simulink library "Hydraulic_Actuator_Lib"  (Simulink 7.9)
settings: Solver=ode45  StartTime=0.0  StopTime=10.0  RelTol=1e-3
undefined symbols (not defined in the file or in its folder): WT_Params
libraries: fl_lib x20, nesl_utility x10, sh_lib x9, mblibv1 x1
Description:
  | Copyright 2011 MathWorks, Inc.
settings Model: Creator=smiller  LastModifiedBy=smiller

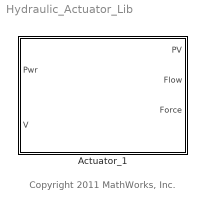
== system Hydraulic_Actuator_Lib ==
  note: Copyright 2011 MathWorks, Inc.
  Actuator_1 : Subsystem
      mask Display: image(imread('Pitch_Hydraulic_Actuator_IMAGE.jpg'));

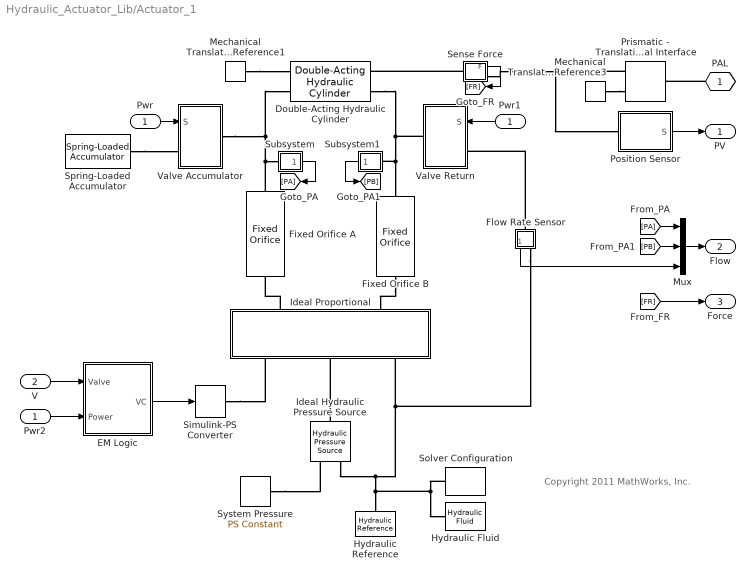
== system Hydraulic_Actuator_Lib/Actuator_1 ==
  note: Copyright 2011 MathWorks, Inc.
  Pwr : Inport
  V : Inport  Port=2
  Double-Acting Hydraulic Cylinder : sh_lib/Hydraulic Cylinders/Double-Acting Hydraulic Cylinder  SystemSampleTime=-1  area_A=WT_Params.Pitch_Actuator.Cylinder.piston_area m^2  area_B=WT_Params.Pitch_Actuator.Cylinder.piston_area m^2  stroke=WT_Params.Pitch_Actuator.Cylinder.stroke m  init_pos=WT_Params.Pitch_Actuator.Cylinder.initial_disp_from_a m  dead_vol_A=1e-04 m^3  dead_vol_B=1e-04 m^3  init_pressure_A=0 Pa  init_pressure_B=0 Pa  k_sh=1.4  stiff=WT_Params.Pitch_Actuator.Cylinder.contact_stiffness N/m  D=WT_Params.Pitch_Actuator.Cylinder.contact_damping N/(m/s)  or=2  LocalVarLogging=[]
  EM Logic : Subsystem
  Fixed Orifice A : sh_lib/Orifices/Fixed Orifice  SystemSampleTime=-1  area=WT_Params.Pitch_Actuator.orifice_area m^2  C_d=0.7  Re_cr=12  flow_rate_Log=off  pr_drop_Log=off  Re_Log=off  power_Log=off  LocalVarNames=|flow_rate|pr_drop|Re|power  LocalVarDescs=|Flow rate through the orifice (m^3/s)|Pressure drop across the orifice (Pa)|Reynolds number|Power (W)  LocalVarLogging=[0 0 0 0]
  Fixed Orifice B : sh_lib/Orifices/Fixed Orifice  SystemSampleTime=-1  area=WT_Params.Pitch_Actuator.orifice_area m^2  C_d=0.7  Re_cr=12  flow_rate_Log=off  pr_drop_Log=off  Re_Log=off  power_Log=off  LocalVarNames=|flow_rate|pr_drop|Re|power  LocalVarDescs=|Flow rate through the orifice (m^3/s)|Pressure drop across the orifice (Pa)|Reynolds number|Power (W)  LocalVarLogging=[0 0 0 0]
  Flow Rate Sensor : Subsystem
      mask Display: disp('F')
  Hydraulic Reference : fl_lib/Hydraulic/Hydraulic Elements/Hydraulic Reference  SystemSampleTime=-1  q_Log=off  LocalVarNames=|q  LocalVarDescs=|q  LocalVarLogging=[]
  Hydraulic Fluid : sh_lib/Hydraulic Utilities/Hydraulic Fluid  SystemSampleTime=-1  DataSource=1  SelFluid=1  SysTemp=60 c  TrapAir=0.005  ViscDerFactor=1  LocalVarLogging=[]
  Ideal Proportional : Subsystem
      mask Display:
      | plot([198.418507352471;198.418507352471], [5.66910021007061;25.5109509453177])
      | plot([189.914857037365;206.922157667577], [25.5109509453177;25.5109509453177])
      | plot([240.936758928001;240.936758928001], [5.66910021007061;25.5109509453177])
      | plot([232.433108612895;249.440409243107], [25.5109509453177;25.5109509453177])
      | plot([240.936758928001;240.936758928001], [76.5328528359532;56.6910021007061])
      | plot([232.433108612895;249.440409243107], [56.6910021007061;56.6910021007061])
      | plot([198.418507352471;198.418507352471], [76.5328528359532;56.6910021007061])
      | plot([189.914857037365;206.922157667577], [56.6910021007061;56.6910021007061])
      | plot([99.2092536762357;99.2092536762357], [76.5328528359532;5.66910021007061])
      | plot([141.727505251765;141.727505251765], [76.5328528359532;5.66910021007061])
      | plot([170.073006302118;170.073006302118], [76.5328528359532;5.66910021007061])
      | plot([269.282259978354;269.282259978354], [76.5328528359532;5.66910021007061])
      | patch([99.2092536762357;93.5401534661651;104.878353886306;99.2092536762357], [76.5328528359532;53.8564519956708;53.8564519956708;76.5328528359532],[0 0 0])
      | plot([99.2092536762357;93.5401534661651;104.878353886306;99.2092536762357], [76.5328528359532;53.8564519956708;53.8564519956708;76.5328528359532])
      | patch([141.727505251765;136.058405041695;147.396605461836;141.727505251765], [5.66910021007061;28.3455010503531;28.3455010503531;5.66910021007061],[0 0 0])
      | plot([141.727505251765;136.058405041695;147.396605461836;141.727505251765], [5.66910021007061;28.3455010503531;28.3455010503531;5.66910021007061])
      | plot([297.627761028707;340.146012604237], [5.66910021007061;76.5328528359532])
      | plot([297.627761028707;340.146012604237], [76.5328528359532;5.66910021007061])
      | plot([70.8637526258826;368.49151365459;368.49151365459;70.8637526258826;70.8637526258826], [76.5328528359532;76.5328528359532;5.66910021007061;5.66910021007061;76.5328528359532])
      | patch([297.627761028707;303.296861238778;311.800511553884;297.627761028707], [5.66910021007061;25.5109509453177;19.8418507352471;5.66910021007061],[0 0 0])
      | plot([297.627761028707;303.296861238778;311.800511553884;297.627761028707], [5.66910021007061;25.5109509453177;19.8418507352471;5.66910021007061])
      | patch([297.627761028707;303.296861238778;311.800511553884;297.627761028707], [76.5328528359532;56.6910021007061;62.3601023107767;76.5328528359532],[0 0 0])
      | plot([297.627761028707;303.296861238778;311.800511553884;297.627761028707], [76.5328528359532;56.6910021007061;62.3601023107767;76.5328528359532])
      | plot([62.3601023107767;374.16061386466], [82.2019530460238;82.2019530460238])
      | plot([65.194652415812;376.995163969696], [0;0])
      | plot([70.8637526258826;0;0;70.8637526258826;70.8637526258826], [53.8564519956708;53.8564519956708;25.5109509453177;25.5109509453177;53.8564519956708]-25.5109509453177+5.66910021007061)
      | plot([70.8637526258826;0;0;70.8637526258826;70.8637526258826]+368.49151365459, [53.8564519956708;53.8564519956708;25.5109509453177;25.5109509453177;53.8564519956708]-25.5109509453177+5.66910021007061)
      | plot([15 25], [5.66910021007061 35])
      | plot([25 15]+405, [5.66910021007061 35])
      | plot([42.5 40]+5,[70 58]);
      | plot([45 50]+2.5,[70 45]);
      | plot([45 50]+7.5,[45 70]);
      | plot([45 50]+12.5,[70 45]);
      | plot([45 50]+17.5,[45 70]);
      | plot([40 42.5]+27.5,[70 58]);
      | plot([42.5 40]+5+324,[70 58]);
      | plot([45 50]+2.5+324,[70 45]);
      | plot([45 50]+7.5+324,[45 70]);
      | plot([45 50]+12.5+324,[70 45]);
      | plot([45 50]+17.5+324,[45 70]);
      | plot([40 42.5]+27.5+324,[70 58]);
      | ;color('red');
      | port_label('LConn', 1,'A')
      | port_label('LConn', 2,'B')
      | port_label('RConn', 1,'S')
      | port_label('RConn', 2,'P')
      | port_label('RConn', 3,'T')
  Ideal Hydraulic Pressure Source : fl_lib/Hydraulic/Hydraulic Sources/Hydraulic Pressure Source  SystemSampleTime=-1  q_Log=off  p_Log=off  LocalVarNames=|flow_rate|pr_differential|power  LocalVarDescs=|Flow rate through the source (m^3/s)|Pressure differential across the source (Pa)|Source power (W)  LocalVarLogging=[0 0 0]
  Mechanical Translational Reference1 : fl_lib/Mechanical/Translational Elements/Mechanical Translational Reference  Tag=Factory Generic  SystemSampleTime=-1  f_Log=off  LocalVarNames=|f  LocalVarDescs=|f  LocalVarLogging=[]
  Mechanical Translational Reference3 : fl_lib/Mechanical/Translational Elements/Mechanical Translational Reference  Tag=Factory Generic  SystemSampleTime=-1  f_Log=off  LocalVarNames=|f  LocalVarDescs=|f  LocalVarLogging=[]
  Mux : Mux  Inputs=3
  Position Sensor : Subsystem
      mask Display:
      | plot([25.5109509453177;56.6910021007061;70.8637526258826;96.3747035712004;127.554754726589;155.900255776942;184.245756827295;212.591257877648;235.26765871793;252.274959348142;283.455010503531], [155.900255776942;155.900255776942;110.547454096377;198.418507352471;113.382004201412;198.418507352471;116.216554306448;198.418507352471;113.382004201412;155.900255776942;155.900255776942])
      | plot([155.900255776942;155.900255776942], [266.447709873319;198.418507352471])
      | patch([155.900255776942;170.073006302118;141.727505251765;155.900255776942], [198.418507352471;226.764008402824;226.764008402824;198.418507352471], [0;0;0])
      | plot([155.900255776942;170.073006302118;141.727505251765;155.900255776942], [198.418507352471;226.764008402824;226.764008402824;198.418507352471])
      | ;
      | color('red');
      | port_label('LConn', 1,'R')
      | port_label('output', 1,'P')
  Prismatic - Translational Interface : mblibv1/Interface  Elements/Prismatic - Translational Interface  UpdateFromCAD=off  DialogClass=PrismaticTranslationalInterface  Primitive=P1
  Pwr1 : InportShadow  Port=1
  Pwr2 : InportShadow  Port=1
  Sense Force : Subsystem
      mask Display: disp('F');
  Simulink-PS Converter : nesl_utility/Simulink-PS Converter  SystemSampleTime=-1  PhysicalDomain=network_engine_domain  LeftPortType=input  RightPortType=output  SubClassName=ps_input  Unit=1  AffineConversion=off  InputFilterTimeConstant=.001  UdotUserProvided=0
  Solver Configuration : nesl_utility/Solver Configuration  SystemSampleTime=-1  PhysicalDomain=network_engine_domain  LeftPortType=input  RightPortType=generic  SubClassName=solver  Accelerate=off  Profile=off  ResidualTolerance=WT_Params.Pitch_Actuator.constraint_tol  MaxNonlinIter=12  MaxModeIter=2  DoFixedCost=off  UseLocalSampling=off  DoDC=off  LinearAlgebra=Sparse  LocalSolverSampleTime=.001  LocalSolverChoice=NE_BACKWARD_EULER_ADVANCER  UseLocalSolver=off
  Spring-Loaded Accumulator : sh_lib/Accumulators/Spring-Loaded Accumulator  SystemSampleTime=-1  capacity=WT_Params.Pitch_Actuator.Accumulator.capacity m^3  pr_preload=WT_Params.Pitch_Actuator.Accumulator.preload_pressure Pa  pr_max=WT_Params.Pitch_Actuator.Accumulator.maximum_pressure Pa  v_init=WT_Params.Pitch_Actuator.Accumulator.initial_volume m^3  str_compl=4e-15 m^3/Pa  flow_rate_Log=off  pr_fluid_Log=off  fluid_volume_Log=off  LocalVarNames=|flow_rate|pr_fluid|fluid_volume  LocalVarDescs=|Accumulator flow rate (m^3/s)|Fluid pressure (Pa)|Initial fluid volume (m^3)  LocalVarLogging=[0 0 0]
  Subsystem : Subsystem
      mask Display: disp('P')
  Subsystem1 : Subsystem
      mask Display: disp('P')
  System Pressure : fl_lib/Physical Signals/Sources/PS Constant  SystemSampleTime=-1  constant=WT_Params.Pitch_Actuator.hydraulic_pressure  LocalVarLogging=[]
  Valve Accumulator : Subsystem
      mask Display:
      | plot([73.6983027309179;124.720204621553], [181.41120672226;181.41120672226])
      | plot([76.2808928266168;277.78591029346], [385.498814284801;385.498814284801])
      | plot([77.0997628569603;276.967040263116], [283.455010503531;283.455010503531])
      | plot([73.6983027309179;276.967040263116;276.967040263116;73.6983027309179;73.6983027309179], [487.542618066072;487.542618066072;79.3674029409885;79.3674029409885;487.542618066072])
      | plot([277.78591029346;226.764008402824], [181.41120672226;181.285226717591])
      | plot([226.764008402824;226.764008402824], [205.28441760689;157.286035828292])
      | patch([206.35524764657;206.35524764657;280.368500389159;206.35524764657], [400.805384851992;370.192243717611;385.498814284801;400.805384851992], [0;0;0])
      | plot([206.35524764657;206.35524764657;280.368500389159;206.35524764657], [400.805384851992;370.192243717611;385.498814284801;400.805384851992])
      | plot([124.720204621553;124.720204621553], [204.906477592885;156.971085816622])
      | plot([0;351.484213024378;351.484213024378;0;0], [566.910021007061;566.910021007061;0;0;566.910021007061])
      | ;
      | color('red');
      | port_label('input', 1,'S');
      | port_label('lconn', 1,'A');
      | port_label('rconn', 1,'B');
  Valve Return : Subsystem
      mask Display:
      | plot([73.6983027309179;124.720204621553], [181.41120672226;181.41120672226])
      | plot([76.2808928266168;277.78591029346], [385.498814284801;385.498814284801])
      | plot([77.0997628569603;276.967040263116], [283.455010503531;283.455010503531])
      | plot([73.6983027309179;276.967040263116;276.967040263116;73.6983027309179;73.6983027309179], [487.542618066072;487.542618066072;79.3674029409885;79.3674029409885;487.542618066072])
      | plot([277.78591029346;226.764008402824], [181.41120672226;181.285226717591])
      | plot([226.764008402824;226.764008402824], [205.28441760689;157.286035828292])
      | patch([206.35524764657;206.35524764657;280.368500389159;206.35524764657], [400.805384851992;370.192243717611;385.498814284801;400.805384851992], [0;0;0])
      | plot([206.35524764657;206.35524764657;280.368500389159;206.35524764657], [400.805384851992;370.192243717611;385.498814284801;400.805384851992])
      | plot([124.720204621553;124.720204621553], [204.906477592885;156.971085816622])
      | plot([0;351.484213024378;351.484213024378;0;0], [566.910021007061;566.910021007061;0;0;566.910021007061])
      | ;
      | color('red');
      | port_label('input', 1,'S');
      | port_label('lconn', 1,'A');
      | port_label('rconn', 1,'B');
  PAL : PMIOPort  Tag=PMCPort  Port=1  Side=Right
  PV : Outport
  Flow : Outport  Port=2
  Force : Outport  Port=3
  wires:
  Pwr2/1 -> EM Logic/2(Power)
  EM Logic/1(VC) -> Simulink-PS Converter/1
  [PB] -> Mux/2
  [PA] -> Mux/1
  Flow Rate Sensor/1(Flow) -> Mux/3
  Subsystem1/1(P) -> [PB]
  Subsystem/1(P) -> [PA]
  V/1 -> EM Logic/1(Valve)
  Pwr1/1 -> Valve Return/1(S)
  Pwr/1 -> Valve Accumulator/1(S)
  Position Sensor/1(S) -> PV/1
  Mux/1 -> Flow/1
  Sense Force/1(F) -> [FR]
  [FR] -> Force/1
  connections:
  Flow Rate Sensor/LConn1 -- Valve Return/LConn1
  Prismatic - Translational Interface/LConn1 -- Position Sensor/LConn1 -- Sense Force/RConn1
  Spring-Loaded Accumulator/RConn1 -- Valve Accumulator/LConn1
  Mechanical Translational Reference1/LConn1 -- Double-Acting Hydraulic Cylinder/LConn1
  Subsystem/LConn1 -- Valve Accumulator/RConn1 -- Double-Acting Hydraulic Cylinder/LConn2 -- Fixed Orifice A/RConn1
  Subsystem1/LConn1 -- Fixed Orifice B/RConn1 -- Valve Return/RConn1 -- Double-Acting Hydraulic Cylinder/RConn2
  Ideal Proportional/LConn1 -- Fixed Orifice A/LConn1
  Fixed Orifice B/LConn1 -- Ideal Proportional/LConn2
  Ideal Proportional/RConn3 -- Flow Rate Sensor/RConn1 -- Hydraulic Reference/LConn1 -- Hydraulic Fluid/RConn1 -- Solver Configuration/RConn1 -- Ideal Hydraulic Pressure Source/RConn2
  Simulink-PS Converter/RConn1 -- Ideal Proportional/RConn1
  Ideal Hydraulic Pressure Source/LConn1 -- Ideal Proportional/RConn2
  System Pressure/RConn1 -- Ideal Hydraulic Pressure Source/RConn1
  Mechanical Translational Reference3/LConn1 -- Prismatic - Translational Interface/LConn2
  PAL/RConn1 -- Prismatic - Translational Interface/RConn1
  Sense Force/LConn1 -- Double-Acting Hydraulic Cylinder/RConn1

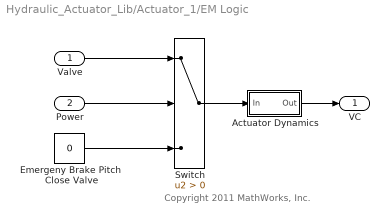
== system Hydraulic_Actuator_Lib/Actuator_1/EM Logic ==
  note: Copyright 2011 MathWorks, Inc.
  Valve : Inport
  Power : Inport  Port=2
  Actuator Dynamics : Subsystem  mask(First-order lag supporting vector signals){b=WT_Params.Pitch_Actuator.hydraulic_actuator_time_constant, x_initial=0}
      mask prompts: b "Filter time constant"; x_initial "Initial output"
      mask help: Models a lag of the form 1/(b*s+1) where s is the Laplace operator.
  Emergeny Brake Pitch  Close Valve : Constant  Value=0
  Switch : Switch  Criteria=u2 > Threshold
  VC : Outport
  wires:
  Switch/1 -> Actuator Dynamics/1(In)
  Emergeny Brake Pitch  Close Valve/1 -> Switch/3
  Power/1 -> Switch/2
  Valve/1 -> Switch/1
  Actuator Dynamics/1(Out) -> VC/1

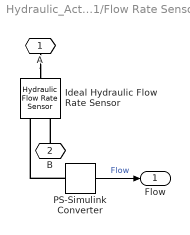
== system Hydraulic_Actuator_Lib/Actuator_1/Flow Rate Sensor ==
  Ideal Hydraulic Flow Rate Sensor : fl_lib/Hydraulic/Hydraulic Sensors/Hydraulic Flow Rate Sensor  SystemSampleTime=-1  q_Log=off  p_Log=off  LocalVarNames=|q|p  LocalVarDescs=|q|p  LocalVarLogging=[]
  PS-Simulink Converter : nesl_utility/PS-Simulink Converter  SystemSampleTime=-1  PhysicalDomain=network_engine_domain  LeftPortType=input  RightPortType=output  SubClassName=ps_output  Unit=1  AffineConversion=off
  A : PMIOPort  Port=1  Side=Left
  B : PMIOPort  Port=2  Side=Right
  Flow : Outport
  wires:
  PS-Simulink Converter/1 -> Flow/1  "Flow"
  connections:
  B/RConn1 -- Ideal Hydraulic Flow Rate Sensor/RConn2
  A/RConn1 -- Ideal Hydraulic Flow Rate Sensor/LConn1
  PS-Simulink Converter/LConn1 -- Ideal Hydraulic Flow Rate Sensor/RConn1

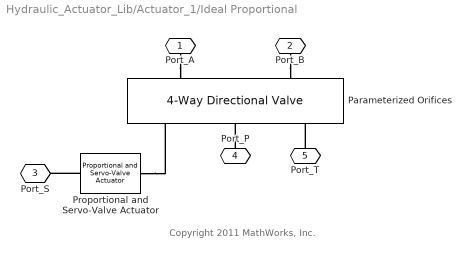
== system Hydraulic_Actuator_Lib/Actuator_1/Ideal Proportional ==
  note: Copyright 2011 MathWorks, Inc.
  Parameterized Orifices : sh_lib/Valves/Directional Valves/4-Way Directional Valve  SystemSampleTime=-1  mdl_type=1  area_max=WT_Params.Pitch_Actuator.Valve.max_area m^2  opening_max=WT_Params.Pitch_Actuator.Valve.max_opening m  opening_tab="[  -0.002 0 0.002 0.005 0.015 ] m"  area_tab="[  1e-09 2.0352e-07 4.0736e-05 0.00011438 0.00034356 ] m^2"  pressure_tab="[  -1e+07 -5e+06 -2e+06 2e+06 5e+06 1e+07 ] Pa"  flow_rate_tab="[  -1e-07 -7.0711e-08 -4.4721e-08 4.4721e-08 7.0711e-08 1e-07 ; -2.0352e-05 -1.4391e-05 -9.1017e-06 9.1017e-06 1.4391e-05 2.0352e-05 ; -0.0040736 -0.0028805 -0.0018218 0.0018218 0.0028805 0.0040736 ; -0.011438 -0.0080879 -0.0051152 0.0051152 0.0080879 0.011438 ; -0.034356 -0.024293 -0.015364 0.015364 0.024293 0.034356 ; ] m^3/s"  interp_method=1  extrap_method=1  C_d=0.7  x_0_P_A=WT_Params.Pitch_Actuator.Valve.initial_opening_pa m  x_0_P_B=WT_Params.Pitch_Actuator.Valve.initial_opening_pb m  x_0_A_T=WT_Params.Pitch_Actuator.Valve.initial_opening_at m  x_0_B_T=WT_Params.Pitch_Actuator.Valve.initial_opening_bt m  Re_cr=12  A_leak=WT_Params.Pitch_Actuator.Valve.leakage_area m^2  LocalVarLogging=[]
  Proportional and Servo-Valve Actuator : sh_lib/Valves/Valve Actuators/Proportional and Servo-Valve Actuator  SystemSampleTime=-1  gain=WT_Params.Pitch_Actuator.Servo.gain  time_constant=WT_Params.Pitch_Actuator.Servo.time_constant s  saturation=WT_Params.Pitch_Actuator.Servo.saturation  LocalVarLogging=[]
  Port_A : PMIOPort  Port=1  Side=Left
  Port_B : PMIOPort  Port=2  Side=Left
  Port_S : PMIOPort  Port=3  Side=Right
  Port_P : PMIOPort  Port=4  Side=Right
  Port_T : PMIOPort  Port=5  Side=Right
  connections:
  Port_A/RConn1 -- Parameterized Orifices/LConn1
  Port_B/RConn1 -- Parameterized Orifices/LConn2
  Proportional and Servo-Valve Actuator/RConn1 -- Parameterized Orifices/RConn1
  Port_P/RConn1 -- Parameterized Orifices/RConn2
  Port_T/RConn1 -- Parameterized Orifices/RConn3
  Proportional and Servo-Valve Actuator/LConn1 -- Port_S/RConn1

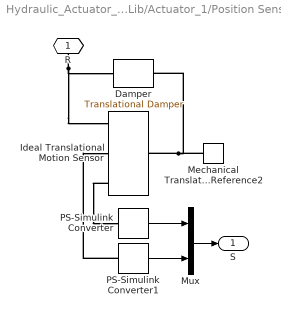
== system Hydraulic_Actuator_Lib/Actuator_1/Position Sensor ==
  Damper : fl_lib/Mechanical/Translational Elements/Translational Damper  SystemSampleTime=-1  D=WT_Params.Pitch_Actuator.Cylinder.damping N/(m/s)  f_Log=off  v_Log=off  LocalVarNames=|force|rel_velocity|power  LocalVarDescs=|Damping force (N)|Damper relative velocity (m/s)|Power dissipated in the damper (W)  LocalVarLogging=[0 0 0]
  Ideal Translational Motion Sensor : fl_lib/Mechanical/Mechanical Sensors/Ideal Translational Motion Sensor  SystemSampleTime=-1  offset=WT_Params.Pitch_Actuator.Sensor.initial_position m  v_Log=off  f_Log=off  x_Log=off  LocalVarNames=|v|f|x  LocalVarDescs=|v|f|x  LocalVarLogging=[]
  Mechanical Translational Reference2 : fl_lib/Mechanical/Translational Elements/Mechanical Translational Reference  Tag=Factory Generic  SystemSampleTime=-1  f_Log=off  LocalVarNames=|f  LocalVarDescs=|f  LocalVarLogging=[]
  Mux : Mux  Inputs=2
  PS-Simulink Converter : nesl_utility/PS-Simulink Converter  SystemSampleTime=-1  PhysicalDomain=network_engine_domain  LeftPortType=input  RightPortType=output  SubClassName=ps_output  Unit=1  AffineConversion=off
  PS-Simulink Converter1 : nesl_utility/PS-Simulink Converter  SystemSampleTime=-1  PhysicalDomain=network_engine_domain  LeftPortType=input  RightPortType=output  SubClassName=ps_output  Unit=1  AffineConversion=off
  R : PMIOPort  Port=1  Side=Left
  S : Outport
  wires:
  PS-Simulink Converter1/1 -> Mux/2
  Mux/1 -> S/1
  PS-Simulink Converter/1 -> Mux/1
  connections:
  PS-Simulink Converter1/LConn1 -- Ideal Translational Motion Sensor/RConn2
  Ideal Translational Motion Sensor/RConn3 -- PS-Simulink Converter/LConn1
  Mechanical Translational Reference2/LConn1 -- Damper/RConn1 -- Ideal Translational Motion Sensor/LConn1
  R/RConn1 -- Damper/LConn1 -- Ideal Translational Motion Sensor/RConn1

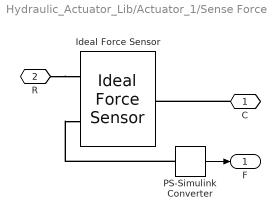
== system Hydraulic_Actuator_Lib/Actuator_1/Sense Force ==
  Ideal Force Sensor : fl_lib/Mechanical/Mechanical Sensors/Ideal Force Sensor  SystemSampleTime=-1  v_Log=off  f_Log=off  LocalVarNames=|v|f  LocalVarDescs=|v|f  LocalVarLogging=[]
  PS-Simulink Converter : nesl_utility/PS-Simulink Converter  SystemSampleTime=-1  PhysicalDomain=network_engine_domain  LeftPortType=input  RightPortType=output  SubClassName=ps_output  Unit=1  AffineConversion=off
  C : PMIOPort  Port=1  Side=Right
  R : PMIOPort  Port=2  Side=Left
  F : Outport
  wires:
  PS-Simulink Converter/1 -> F/1
  connections:
  PS-Simulink Converter/LConn1 -- Ideal Force Sensor/RConn2
  C/RConn1 -- Ideal Force Sensor/LConn1
  R/RConn1 -- Ideal Force Sensor/RConn1

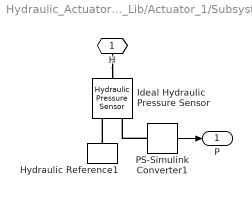
== system Hydraulic_Actuator_Lib/Actuator_1/Subsystem ==
  Hydraulic Reference1 : fl_lib/Hydraulic/Hydraulic Elements/Hydraulic Reference  SystemSampleTime=-1  q_Log=off  LocalVarNames=|q  LocalVarDescs=|q  LocalVarLogging=[]
  Ideal Hydraulic Pressure Sensor : fl_lib/Hydraulic/Hydraulic Sensors/Hydraulic Pressure Sensor  SystemSampleTime=-1  q_Log=off  p_Log=off  LocalVarNames=|q|p  LocalVarDescs=|q|p  LocalVarLogging=[]
  PS-Simulink Converter1 : nesl_utility/PS-Simulink Converter  SystemSampleTime=-1  PhysicalDomain=network_engine_domain  LeftPortType=input  RightPortType=output  SubClassName=ps_output  Unit=1  AffineConversion=off
  H : PMIOPort  Port=1  Side=Left
  P : Outport
  wires:
  PS-Simulink Converter1/1 -> P/1
  connections:
  H/RConn1 -- Ideal Hydraulic Pressure Sensor/LConn1
  PS-Simulink Converter1/LConn1 -- Ideal Hydraulic Pressure Sensor/RConn2
  Hydraulic Reference1/LConn1 -- Ideal Hydraulic Pressure Sensor/RConn1

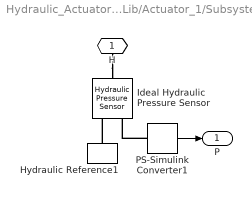
== system Hydraulic_Actuator_Lib/Actuator_1/Subsystem1 ==
  Hydraulic Reference1 : fl_lib/Hydraulic/Hydraulic Elements/Hydraulic Reference  SystemSampleTime=-1  q_Log=off  LocalVarNames=|q  LocalVarDescs=|q  LocalVarLogging=[]
  Ideal Hydraulic Pressure Sensor : fl_lib/Hydraulic/Hydraulic Sensors/Hydraulic Pressure Sensor  SystemSampleTime=-1  q_Log=off  p_Log=off  LocalVarNames=|q|p  LocalVarDescs=|q|p  LocalVarLogging=[]
  PS-Simulink Converter1 : nesl_utility/PS-Simulink Converter  SystemSampleTime=-1  PhysicalDomain=network_engine_domain  LeftPortType=input  RightPortType=output  SubClassName=ps_output  Unit=1  AffineConversion=off
  H : PMIOPort  Port=1  Side=Left
  P : Outport
  wires:
  PS-Simulink Converter1/1 -> P/1
  connections:
  Hydraulic Reference1/LConn1 -- Ideal Hydraulic Pressure Sensor/RConn1
  PS-Simulink Converter1/LConn1 -- Ideal Hydraulic Pressure Sensor/RConn2
  H/RConn1 -- Ideal Hydraulic Pressure Sensor/LConn1

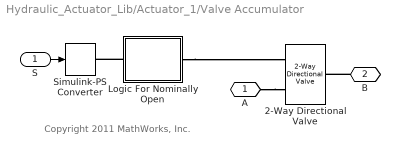
== system Hydraulic_Actuator_Lib/Actuator_1/Valve Accumulator ==
  note: Copyright 2011 MathWorks, Inc.
  S : Inport
  2-Way Directional Valve : sh_lib/Valves/Directional Valves/2-Way Directional Valve  SystemSampleTime=-1  mdl_type=1  area_max=WT_Params.Pitch_Actuator.Emergency_Pitch_Valve.max_area m^2  opening_max=0.005 m  opening_tab="[  -0.002 0 0.002 0.005 0.015 ] m"  area_tab="[  1e-09 2.0352e-07 4.0736e-05 0.00011438 0.00034356 ] m^2"  pressure_tab="[  -1e+07 -5e+06 -2e+06 2e+06 5e+06 1e+07 ] Pa"  flow_rate_tab="[  -1e-07 -7.0711e-08 -4.4721e-08 4.4721e-08 7.0711e-08 1e-07 ; -2.0352e-05 -1.4391e-05 -9.1017e-06 9.1017e-06 1.4391e-05 2.0352e-05 ; -0.0040736 -0.0028805 -0.0018218 0.0018218 0.0028805 0.0040736 ; -0.011438 -0.0080879 -0.0051152 0.0051152 0.0080879 0.011438 ; -0.034356 -0.024293 -0.015364 0.015364 0.024293 0.034356 ; ] m^3/s"  interp_method=1  extrap_method=1  C_d=0.7  x_0=0 m  Re_cr=12  A_leak=1e-12 m^2  LocalVarLogging=[]
  Logic For Nominally Open : Subsystem
  Simulink-PS Converter : nesl_utility/Simulink-PS Converter  SystemSampleTime=-1  PhysicalDomain=network_engine_domain  LeftPortType=input  RightPortType=output  SubClassName=ps_input  Unit=1  AffineConversion=off  InputFilterTimeConstant=.001  UdotUserProvided=0
  A : PMIOPort  Port=1  Side=Left
  B : PMIOPort  Port=2  Side=Right
  wires:
  S/1 -> Simulink-PS Converter/1
  connections:
  Logic For Nominally Open/RConn1 -- 2-Way Directional Valve/LConn1
  B/RConn1 -- 2-Way Directional Valve/RConn1
  A/RConn1 -- 2-Way Directional Valve/LConn2
  Logic For Nominally Open/LConn1 -- Simulink-PS Converter/RConn1

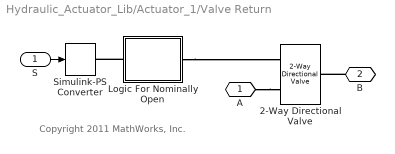
== system Hydraulic_Actuator_Lib/Actuator_1/Valve Return ==
  note: Copyright 2011 MathWorks, Inc.
  S : Inport
  2-Way Directional Valve : sh_lib/Valves/Directional Valves/2-Way Directional Valve  SystemSampleTime=-1  mdl_type=1  area_max=WT_Params.Pitch_Actuator.Emergency_Pitch_Valve.max_area m^2  opening_max=0.005 m  opening_tab="[  -0.002 0 0.002 0.005 0.015 ] m"  area_tab="[  1e-09 2.0352e-07 4.0736e-05 0.00011438 0.00034356 ] m^2"  pressure_tab="[  -1e+07 -5e+06 -2e+06 2e+06 5e+06 1e+07 ] Pa"  flow_rate_tab="[  -1e-07 -7.0711e-08 -4.4721e-08 4.4721e-08 7.0711e-08 1e-07 ; -2.0352e-05 -1.4391e-05 -9.1017e-06 9.1017e-06 1.4391e-05 2.0352e-05 ; -0.0040736 -0.0028805 -0.0018218 0.0018218 0.0028805 0.0040736 ; -0.011438 -0.0080879 -0.0051152 0.0051152 0.0080879 0.011438 ; -0.034356 -0.024293 -0.015364 0.015364 0.024293 0.034356 ; ] m^3/s"  interp_method=1  extrap_method=1  C_d=0.7  x_0=0 m  Re_cr=12  A_leak=1e-12 m^2  LocalVarLogging=[]
  Logic For Nominally Open : Subsystem
  Simulink-PS Converter : nesl_utility/Simulink-PS Converter  SystemSampleTime=-1  PhysicalDomain=network_engine_domain  LeftPortType=input  RightPortType=output  SubClassName=ps_input  Unit=1  AffineConversion=off  InputFilterTimeConstant=.001  UdotUserProvided=0
  A : PMIOPort  Port=1  Side=Left
  B : PMIOPort  Port=2  Side=Right
  wires:
  S/1 -> Simulink-PS Converter/1
  connections:
  Logic For Nominally Open/LConn1 -- Simulink-PS Converter/RConn1
  A/RConn1 -- 2-Way Directional Valve/LConn2
  B/RConn1 -- 2-Way Directional Valve/RConn1
  Logic For Nominally Open/RConn1 -- 2-Way Directional Valve/LConn1

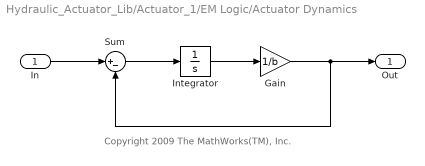
== system Hydraulic_Actuator_Lib/Actuator_1/EM Logic/Actuator Dynamics ==
  note: Copyright 2009 The MathWorks(TM), Inc.
  In : Inport
  Gain : Gain  Gain=1/b
  Integrator : Integrator  InitialCondition=x_initial
  Sum : Sum  Inputs=|+-  SaturateOnIntegerOverflow=on  InputSameDT=on  OutDataTypeStr=Inherit: Same as first input
  Out : Outport
  wires:
  Gain/1 -> Out/1, Sum/2
  Integrator/1 -> Gain/1
  In/1 -> Sum/1
  Sum/1 -> Integrator/1

== system Hydraulic_Actuator_Lib/Actuator_1/Valve Accumulator/Logic For Nominally Open ==
  PS Gain : fl_lib/Physical Signals/Functions/PS Gain  SystemSampleTime=-1  gain=-1  LocalVarLogging=[]
  PS Subtract : fl_lib/Physical Signals/Functions/PS Subtract  SystemSampleTime=-1  LocalVarLogging=[]
  Voltage_Open : fl_lib/Physical Signals/Sources/PS Constant  SystemSampleTime=-1  constant=24  LocalVarLogging=[]
  S : PMIOPort  Port=1  Side=Left
  VA : PMIOPort  Port=2  Side=Right
  connections:
  VA/RConn1 -- PS Gain/RConn1
  S/RConn1 -- PS Subtract/LConn1
  PS Subtract/RConn1 -- PS Gain/LConn1
  PS Subtract/LConn2 -- Voltage_Open/RConn1

== system Hydraulic_Actuator_Lib/Actuator_1/Valve Return/Logic For Nominally Open ==
  PS Gain : fl_lib/Physical Signals/Functions/PS Gain  SystemSampleTime=-1  gain=-1  LocalVarLogging=[]
  PS Subtract : fl_lib/Physical Signals/Functions/PS Subtract  SystemSampleTime=-1  LocalVarLogging=[]
  Voltage_Open : fl_lib/Physical Signals/Sources/PS Constant  SystemSampleTime=-1  constant=24  LocalVarLogging=[]
  S : PMIOPort  Port=1  Side=Left
  VA : PMIOPort  Port=2  Side=Right
  connections:
  PS Subtract/LConn2 -- Voltage_Open/RConn1
  PS Subtract/RConn1 -- PS Gain/LConn1
  S/RConn1 -- PS Subtract/LConn1
  VA/RConn1 -- PS Gain/RConn1
